simulink model "lab6fsf_linear"  (R2024a)
settings: Solver=VariableStepAuto  StartTime=0.0  StopTime=10.0  RelTol=1e-3
values from neighbouring files (symbols this model uses):
  k1 = lqr(A,B,Q,R)    [ica19_runscript.m]
  x0 = [0;0;5/180*pi;0]    [ica19_runscript.m]
  xs = [0;0;0;0]    [ica19_runscript.m]
undefined symbols (not defined in the file or in its folder): A, B
settings Model: Creator=Lauren  LastModifiedBy=Lauren
settings DataIOCC: SaveOutput=off  SignalLogging=off  DSMLogging=off  SaveTime=off  ReturnWorkspaceOutputs=off

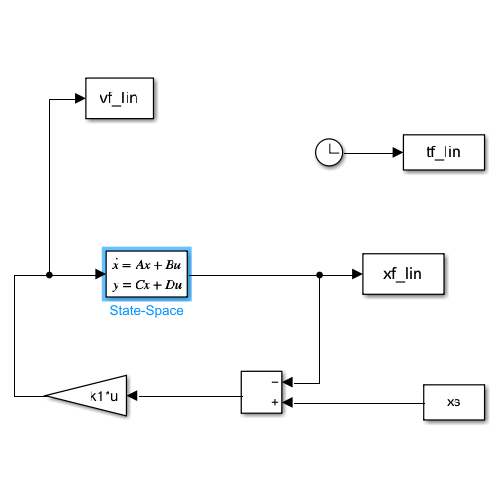
[thumbnail: Simulink's stored preview of the top-level diagram]
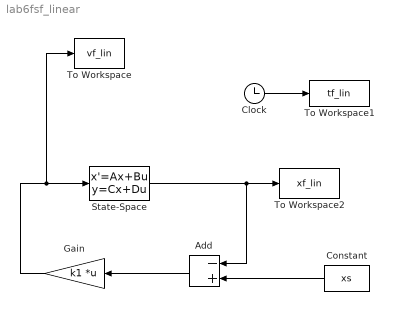
== system lab6fsf_linear ==
  Add : Sum  Inputs=-+
  Clock : Clock
  Constant : Constant  Value=xs
  Gain : Gain  Gain=k1  Multiplication=Matrix(K*u)
  State-Space : StateSpace  A=A  B=B  C=eye(4,4)  D=[0;0;0;0]  InitialCondition=x0
  To Workspace : ToWorkspace  VariableName=vf_lin  SampleTime=-1
      settings: Save2DSignal=2-D array (concatenate along first dimension)
  To Workspace1 : ToWorkspace  VariableName=tf_lin  SampleTime=-1
      settings: Save2DSignal=2-D array (concatenate along first dimension)
  To Workspace2 : ToWorkspace  VariableName=xf_lin  SampleTime=-1
      settings: Save2DSignal=2-D array (concatenate along first dimension)
  wires:
  Clock/1 -> To Workspace1/1
  State-Space/1 -> Add/1, To Workspace2/1
  Add/1 -> Gain/1
  Constant/1 -> Add/2
  Gain/1 -> State-Space/1, To Workspace/1
